simulink model "ysw7_5"  (R2014a)
settings: Solver=ode15s  StartTime=0.0  StopTime=1  RelTol=1e-3
libraries: powerlib x7
settings Model: Creator=Administrator  LastModifiedBy=Administrator

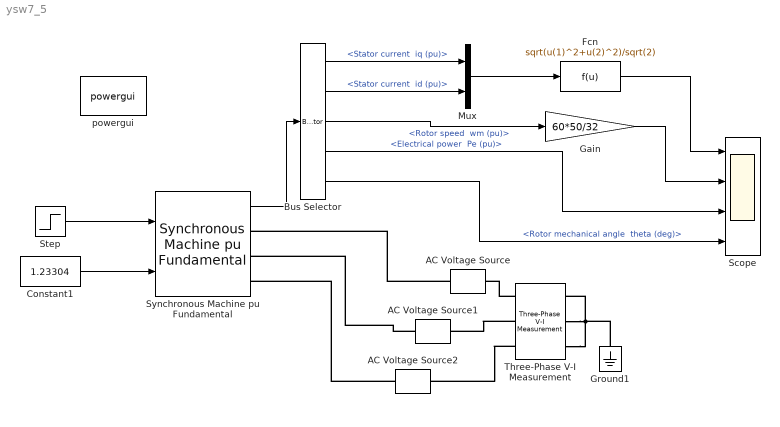
== system ysw7_5 ==
  AC Voltage Source : powerlib/Electrical Sources/AC Voltage Source  Amplitude=100  Phase=0  Frequency=50  SampleTime=0  Measurements=None
  AC Voltage Source1 : powerlib/Electrical Sources/AC Voltage Source  Amplitude=100  Phase=0  Frequency=50  SampleTime=0  Measurements=None
  AC Voltage Source2 : powerlib/Electrical Sources/AC Voltage Source  Amplitude=100  Phase=0  Frequency=50  SampleTime=0  Measurements=None
  Bus Selector : BusSelector  OutputSignals="dq0 components.Stator current  iq (pu),dq0 components.Stator current  id (pu),Mechanical.Rotor speed  wm (pu),Mechanical.Electrical power  Pe (pu),Mechanical.Rotor mechanical angle  theta (deg)"
  Constant1 : Constant  Value=1.23304
  Fcn : Fcn  Expr=sqrt(u(1)^2+u(2)^2)/sqrt(2)
  Gain : Gain  Gain=60*50/32
  Ground1 : powerlib/Elements/Ground  LConnTagsString=a
  Mux : Mux  Inputs=2
  Scope : Scope  NumInputPorts=4
      settings: YMin=-5~-5~-5~-5  YMax=5~5~5~5
  Step : Step  Time=0.6  Before=0.8  After=0.6  SampleTime=0
  Synchronous Machine pu Fundamental : powerlib/Machines/Synchronous Machine pu Fundamental  PresetModel=No  MechanicalLoad=Mechanical power Pm  ShowDetailedParameters=on  RotorType=Salient-pole  Units=per unit fundamental parameters  MeasurementBus=off  NominalParameters="[ 50E6  10.5e3   50]"  Stator="[0.003  0.19837  0.91763  0.21763 ]"  Field="[ 6.3501E-04  0.16537]"  Dampers2=[0.0652, 0.5134, 0.0287, 0.2553, 7.765e-3, 0.9167 ]  Dampers1="[ 4.6454E-03  3.9203e-02  6.8430E-03  1.4544e-02 ]"  Mechanical=[ 3.195 0 32]  PolePairs=20  InitialConditions="[ 0  -71.6365  0.8  0.8  0.8  -0.0279696  -120.02  119.972  1.23304 ]"  SetSaturation=off  Saturation=[0.6404,0.7127,0.8441,0.9214,0.9956,1.082,1.19,1.316,1.457;0.7,0.7698,0.8872,0.9466,0.9969,1.046,1.1,1.151,1.201]  LoadFlowParameters=[1,0,0,0,0]  TsPowergui=0  TsBlock=-1  IterativeModel=Trapezoidal non iterative  BusType=PV  Pref=0  Qref=0  Qmin=-inf  Qmax=inf  PLF=0  QLF=0
  Three-Phase V-I Measurement : powerlib/Measurements/Three-Phase V-I Measurement  VoltageMeasurement=phase-to-ground  SetLabelV=on  LabelV=Vabc  Vpu=on  VpuLL=off  CurrentMeasurement=yes  SetLabelI=on  LabelI=Iabc  Ipu=on  Pbase=100e6  Vbase=500e3  OutputType=Complex  PhasorSimulation=off  PSBequivalent=0
  powergui : powerlib/powergui  Priority=1  SimulationMode=Continuous  SolverType=Tustin  SampleTime=50e-6  frequency=60  SPID=off  DisableSnubberDevices=off  DisableRonSwitches=off  DisableVfSwitches=off  SwTol=0  Interpol=off  DisplayEquations=off  Ts=0  methode=off  frequencyindice=50  Pbase=100e6  ErrMax=1e-4  Iterations=50  UnitsV=kV  UnitsW=MW  FunctionMessages=off  echomessages=off  HookPort=off  EnableUseOfTLC=off  x0status=blocks  RestoreLinks=warning  ResistiveCurrentMeasurement=off  Frange=[0:2:500]  Ylog=off  Xlog=on  ShowGrid=off  save=off  variable=ZData  structure=0  ZoomFFT=off  StartTime=0.0  cycles=1  DisplayStyle=1  fundamental=60  FreqAxis=off  MaxFrequency=1000  frequencyindicesteady=1  RmsSteady=1  display=off
  wires:
  Synchronous Machine pu Fundamental/1 -> Bus Selector/1
  Constant1/1 -> Synchronous Machine pu Fundamental/2
  Step/1 -> Synchronous Machine pu Fundamental/1
  Fcn/1 -> Scope/1
  Bus Selector/5 -> Scope/4  "<Rotor mechanical angle  theta (deg)>"
  Bus Selector/3 -> Gain/1  "<Rotor speed  wm (pu)>"
  Gain/1 -> Scope/2
  Bus Selector/4 -> Scope/3  "<Electrical power  Pe (pu)>"
  Bus Selector/2 -> Mux/2  "<Stator current  id (pu)>"
  Bus Selector/1 -> Mux/1  "<Stator current  iq (pu)>"
  Mux/1 -> Fcn/1
  connections:
  Three-Phase V-I Measurement/RConn2 -- Ground1/LConn1 -- Three-Phase V-I Measurement/RConn1 -- Three-Phase V-I Measurement/RConn3
  Three-Phase V-I Measurement/LConn2 -- AC Voltage Source1/LConn1
  Three-Phase V-I Measurement/LConn1 -- AC Voltage Source/LConn1
  Three-Phase V-I Measurement/LConn3 -- AC Voltage Source2/LConn1
  AC Voltage Source2/RConn1 -- Synchronous Machine pu Fundamental/RConn3
  AC Voltage Source1/RConn1 -- Synchronous Machine pu Fundamental/RConn2
  AC Voltage Source/RConn1 -- Synchronous Machine pu Fundamental/RConn1
